simulink model "SF034A_AssiPahFwl"  (R2013b)
settings: Solver=FixedStepDiscrete  SolverMode=SingleTasking  StartTime=0.0  StopTime=1  FixedStep=0.002  RelTol=1e-3
values from neighbouring files (symbols this model uses):
  ARCHGLBPRM_2MILLISEC_SEC_F32 = DataDict.Constant    [SF034A_AssiPahFwl_DataDict.m]
  AssiPahFwlDiRcvr = DataDict.Calibration    [SF034A_AssiPahFwl_DataDict.m]
  AssiPahFwlHysCmpLim = DataDict.Calibration    [SF034A_AssiPahFwl_DataDict.m]
  AssiPahFwlRestoreThd = DataDict.Calibration    [SF034A_AssiPahFwl_DataDict.m]
  BasAssiPahFwlOverLimDiagcFailStep = DataDict.Calibration    [SF034A_AssiPahFwl_DataDict.m]
  BasAssiPahFwlOverLimDiagcPassStep = DataDict.Calibration    [SF034A_AssiPahFwl_DataDict.m]
  BASASSIREACHED_CNT_U08 = DataDict.Constant    [SF034A_AssiPahFwl_DataDict.m]
  HiFrqAssiPahFwlOverLimDiagcFailStep = DataDict.Calibration    [SF034A_AssiPahFwl_DataDict.m]
  HiFrqAssiPahFwlOverLimDiagcPassStep = DataDict.Calibration    [SF034A_AssiPahFwl_DataDict.m]
  HIFRQASSIREACHED_CNT_U08 = DataDict.Constant    [SF034A_AssiPahFwl_DataDict.m]
undefined symbols (not defined in the file or in its folder): MfgEnaSt1, NtcNr1, NtcSts1, sigbuilder_block, SigQlfr1
libraries: simulink x23, Fil x8, NxtrLim x5, FixdToFloat x5, BilnrIntrpnMplX x4, FloatToFixd x4, NxtrAbslt x2, LnrIntrpn x1, NxtrSign x1
(part 1 of 3)
settings Model: Creator=SNEHAP1  LastModifiedBy=PallavG
settings SolverCC: AutoInsertRateTranBlk=on  InsertRTBMode=Always
settings DataIOCC: LimitDataPoints=off  SaveFormat=Structure  ReturnWorkspaceOutputs=on
settings OptimizationCC: BlockReduction=off  InlineParams=on  ZeroExternalMemoryAtStartup=off  ZeroInternalMemoryAtStartup=off  OptimizeModelRefInitCode=on  LifeSpan=1
settings DebuggingCC: SignalInfNanChecking=error  SignalRangeChecking=warning  UnderspecifiedInitializationDetection=Simplified  SolverPrmCheckMsg=error  InheritedTsInSrcMsg=error  DiscreteInheritContinuousMsg=error  SingleTaskRateTransMsg=error  TasksWithSamePriorityMsg=error  SigSpecEnsureSampleTimeMsg=error  CheckMatrixSingularityMsg=error  ParameterUnderflowMsg=error  ParameterPrecisionLossMsg=error  ParameterTunabilityLossMsg=error  FixptConstUnderflowMsg=warning  FixptConstOverflowMsg=warning  VectorMatrixConversionMsg=error  SignalLabelMismatchMsg=error  UnconnectedInputMsg=error  UnconnectedOutputMsg=error  UnconnectedLineMsg=error  SFcnCompatibilityMsg=error  UniqueDataStoreMsg=warning  BusObjectLabelMismatch=error  RootOutportRequireBusObject=error  AssertControl=DisableAll  ModelReferenceIOMsg=error  ModelReferenceVersionMismatchMessage=warning  ModelReferenceIOMismatchMessage=error  ModelReferenceCSMismatchMessage=warning  ModelReferenceDataLoggingMessage=error  StateNameClashWarn=warning  StrictBusMsg=ErrorOnBusTreatedAsVector  NonBusSignalsTreatedAsBus=error  SFUnexpectedBacktrackingDiag=error  SFInvalidInputDataAccessInChartInitDiag=error  SFNoUnconditionalDefaultTransitionDiag=error  SFTransitionOutsideNaturalParentDiag=error  SFUnconditionalTransitionShadowingDiag=error  SFUndirectedBroadcastEventsDiag=error
settings ModelReferenceCC: ModelReferenceNumInstancesAllowed=Single
settings RTWCC: SystemTargetFile=autosar.tlc  GenCodeOnly=on  TemplateMakefile=ert_default_tmf  Description=AUTOSAR  GenerateReport=on  ProcessScript=autosar_make_rtw_hook  LaunchReport=on
settings CodeAppCC: GenerateComments=off  IgnoreCustomStorageClasses=off  CustomSymbolStrType=$N$R$M  CustomSymbolStrBlkIO=$N$M  SimulinkBlockComments=off
settings STFCustomTargetCC: ParMdlRefBuildCompliant=on  CompOptLevelCompliant=on  IncludeMdlTerminateFcn=off  CombineOutputUpdateFcns=on  SuppressErrorStatus=on  ERTFirstTimeCompliant=on  ERTCustomFileBanners=on  SupportNonFinite=off  SupportComplex=off  SupportContinuousTime=off  SupportNonInlinedSFcns=off  MATLABClassNameForMDSCustomization=Simulink.SoftwareTarget.ERTCustomization  AutosarCompliant=on  GRTInterface=off  SystemTargetFile=autosar.tlc
settings ERTTargetCC: CodeReplacementLibrary=ANSI_C  ConcurrentExecutionCompliant=off  IncludeMdlTerminateFcn=off  SuppressErrorStatus=on  SupportNonFinite=off  SupportComplex=off  ModelStepFunctionPrototypeControlCompliant=off  CPPClassGenCompliant=off  AutosarCompliant=on  InlinedParameterPlacement=NonHierarchical  ERTCustomFileTemplate=example_file_process.tlc  EnableUserReplacementTypes=on

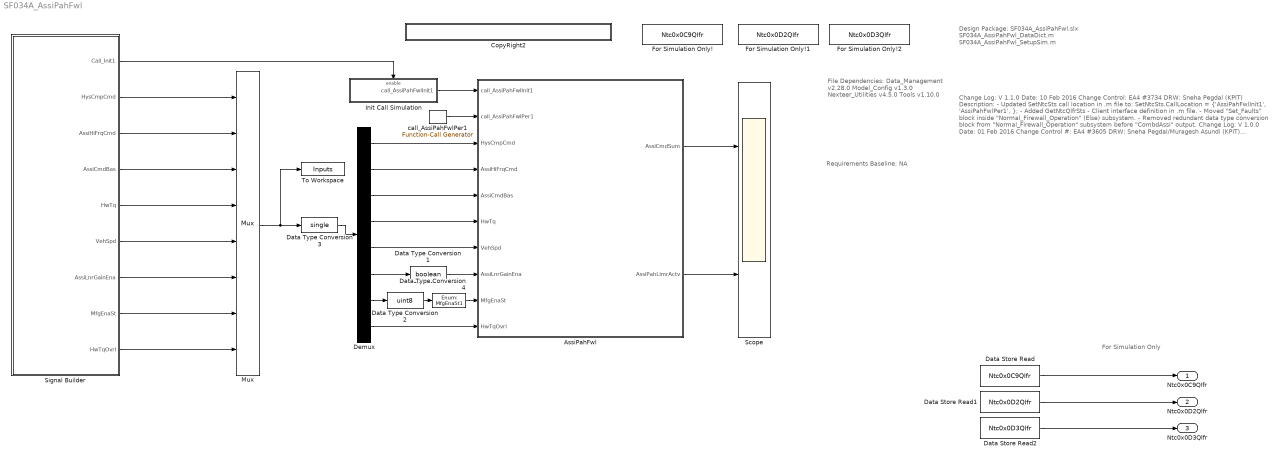
== system SF034A_AssiPahFwl ==
  note: Change Log:  V 1.1.0
      |  Date: 10 Feb 2016
      |  Change Control: EA4 #3734
      |  DRW: Sneha Pegdal (KPIT)
      |  Description:
      | - Updated SetNtcSts call location in .m file to:
      |   SetNtcSts.CallLocation = {'AssiPahFwlInit1', 'AssiPahFwlPer1', };
      | - Added GetNtcQlfrSts - Client interface definition in .m file.
      | - Moved "Set_Faults" block inside "Normal_Firewall_Operation" (Else) subsystem.
      | - Removed redundant data type conversion block from "Normal_Firewall_Operation" subsystem before
      |   "CombdAssi" output.
      |
      |
      |  Change Log:  V 1.0.0
      |  Date: 01 Feb 2016
      |  Change Control #: EA4 #3605
      |  DRW: Sneha Pegdal/Muragesh Asundi (KPIT)
      |  Description:
      |   -Initial Release of EA4 from EA3 V 10.0.0
  note: Requirements Baseline: NA
  note: For Simulation Only
  note: File Dependencies:
      |
      | Data_Management v2.28.0
      | Model_Config v1.3.0
      | Nexteer_Utilities v4.5.0
      | Tools v1.10.0
  note: Design Package:
      |
      | SF034A_AssiPahFwl.slx
      | SF034A_AssiPahFwl_DataDict.m
      | SF034A_AssiPahFwl_SetupSim.m
  AssiPahFwl : Subsystem
  CopyRight2 : Subsystem  Description=|  mask(Copyright Information){none=on}
      | Copyright info block.                                               
      |                                                                     
      | Place copyright information at the top of every subsystem in design.
      mask prompts: none "No parameters"
      mask help: Place copyright information at the top of every subsystem in design.
      mask Display:
      | NxtrConf = 'Nexteer Confidential';
      | 
      | sys = bdroot; %handle for the current model ("system")
      | first = get_param(sys,'Created');
      | first = first(end-3:end);  %year is last four digits
      | 
      | last = get_param(sys,'LastModifiedDate');
      | if isempty(last)
      |     last = datestr(now,'yyyy');
      | else
      |     last = last(end-3:end);
      | end
      | 
      | if strcmp(first,last)
      |     fprintf('%s -- Copyright %s Nexteer',NxtrConf,first)
      | else
      |     fprintf('%s -- %s%s- %s Nexteer',NxtrConf,char(169),first,last)
      | end
  Data Store Read : DataStoreRead  DataStoreName=Ntc0x0C9Qlfr  SampleTime=.002
  Data Store Read1 : DataStoreRead  DataStoreName=Ntc0x0D2Qlfr  SampleTime=.002
  Data Store Read2 : DataStoreRead  DataStoreName=Ntc0x0D3Qlfr  SampleTime=.002
  Data Type Conversion1 : DataTypeConversion  OutDataTypeStr=boolean
  Data Type Conversion2 : DataTypeConversion  OutDataTypeStr=uint8
  Data Type Conversion3 : DataTypeConversion  OutDataTypeStr=single
  Data Type Conversion4 : DataTypeConversion  OutDataTypeStr=Enum: MfgEnaSt1
  Demux : Demux  Outputs=8
  For Simulation Only! : DataStoreMemory  DataStoreName=Ntc0x0C9Qlfr  InitialValue=SigQlfr1.SIGQLFR_NORES  OutDataTypeStr=Enum: SigQlfr1
  For Simulation Only!1 : DataStoreMemory  DataStoreName=Ntc0x0D2Qlfr  InitialValue=SigQlfr1.SIGQLFR_NORES  OutDataTypeStr=Enum: SigQlfr1
  For Simulation Only!2 : DataStoreMemory  DataStoreName=Ntc0x0D3Qlfr  InitialValue=SigQlfr1.SIGQLFR_NORES  OutDataTypeStr=Enum: SigQlfr1
  Init Call Simulation : Subsystem  TreatAsAtomicUnit=on
  Mux : Mux  Inputs=8
  Scope : Scope  NumInputPorts=2
      settings: YMin=-5~-5  YMax=5~5
  Signal Builder : Subsystem  Tag=STV Subsys  LoadFcn=sigbuilder_block('load');  StartFcn=sigbuilder_block('start');  StopFcn=sigbuilder_block('stop');  ClipboardFcn=sigbuilder_block('clipboard');  mask(Sigbuilder block){}
      mask help: Simulink:masks:SigbuilderBlock_MD
      mask init:
      | if ~strcmp(get_param(bdroot(gcbh),'SimulationStatus'),'stopped') tuvar = sigbuilder_block('maskInit'); end
      settings: CopyFcn=sigbuilder_block('copy');  DeleteFcn=sigbuilder_block('delete');  ModelCloseFcn=sigbuilder_block('modelClose');  PreSaveFcn=sigbuilder_block('preSave');  PauseFcn=sigbuilder_block('pause');  ContinueFcn=sigbuilder_block('continue');  NameChangeFcn=sigbuilder_block('namechange');  OpenFcn=sigbuilder_block('open',[6 28.5 756 480 ]);  CloseFcn=sigbuilder_block('close');
      mask Display: plot(0, 0, 100, 100,[2, 2, 32, 32, 2], [68, 8, 8, 68, 68],[32, 2], [38, 38], [32, 19, 2],[53, 60, 44], [32, 17, 17, 2],[16, 16, 31, 31]);txt = getActiveGroup(gcbh);text(2, 100, txt,'verticalAlignment', 'top');
  To Workspace : ToWorkspace  VariableName=Inputs  SampleTime=-1
  call_AssiPahFwlPer1 : simulink/Ports & Subsystems/Function-Call Generator  RequirementInfo={} %GIDa_9fbb524b_78b2_48c0_ad45_2c0b0cc0a9b8  sample_time=0.002  numberOfIterations=1
  Ntc0x0C9Qlfr : Outport
  Ntc0x0D2Qlfr : Outport  Port=2
  Ntc0x0D3Qlfr : Outport  Port=3
  wires:
  call_AssiPahFwlPer1/1 -> AssiPahFwl/2(call_AssiPahFwlPer1)
  Data Store Read/1 -> Ntc0x0C9Qlfr/1
  Data Store Read1/1 -> Ntc0x0D2Qlfr/1
  Data Store Read2/1 -> Ntc0x0D3Qlfr/1
  Mux/1 -> Data Type Conversion3/1, To Workspace/1
  Init Call Simulation/1(call_AssiPahFwlInit1) -> AssiPahFwl/1(call_AssiPahFwlInit1)
  Demux/3 -> AssiPahFwl/5(AssiCmdBas)
  Demux/4 -> AssiPahFwl/6(HwTq)
  Demux/2 -> AssiPahFwl/4(AssiHiFrqCmd)
  Demux/5 -> AssiPahFwl/7(VehSpd)
  Demux/1 -> AssiPahFwl/3(HysCmpCmd)
  Demux/7 -> Data Type Conversion2/1
  Demux/8 -> AssiPahFwl/10(HwTqOvrl)
  AssiPahFwl/1(AssiCmdSum) -> Scope/1
  AssiPahFwl/2(AssiPahLimrActv) -> Scope/2
  Signal Builder/1(Call_Init1) -> Init Call Simulation/Enable
  Signal Builder/2(HysCmpCmd) -> Mux/1
  Signal Builder/3(AssiHiFrqCmd) -> Mux/2
  Signal Builder/4(AssiCmdBas) -> Mux/3
  Signal Builder/5(HwTq) -> Mux/4
  Signal Builder/6(VehSpd) -> Mux/5
  Signal Builder/7(AssiLnrGainEna) -> Mux/6
  Signal Builder/8(MfgEnaSt) -> Mux/7
  Signal Builder/9(HwTqOvrl) -> Mux/8
  Data Type Conversion3/1 -> Demux/1
  Demux/6 -> Data Type Conversion1/1
  Data Type Conversion1/1 -> AssiPahFwl/8(AssiLnrGainEna)
  Data Type Conversion2/1 -> Data Type Conversion4/1
  Data Type Conversion4/1 -> AssiPahFwl/9(MfgEnaSt)

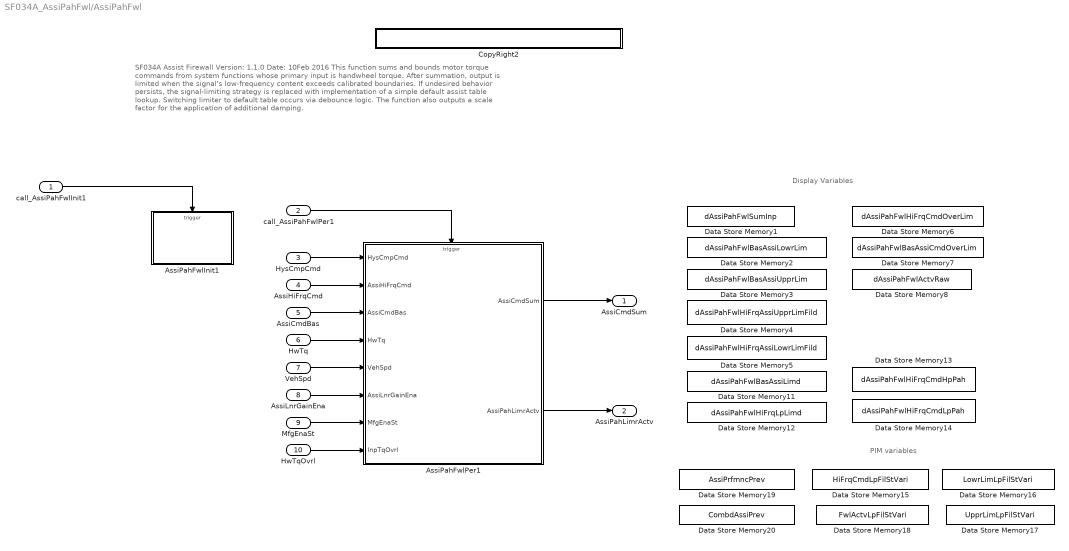
== system SF034A_AssiPahFwl/AssiPahFwl ==
  note: Display Variables
  note: SF034A Assist Firewall
      | Version: 1.1.0                                                                                                                                                                                           Date: 10Feb 2016
      |
      | This function sums and bounds motor torque commands from system functions whose primary input is handwheel torque.
      | After summation, output is limited when the signal's low-frequency content
      | exceeds calibrated boundaries.  If undesired behavior persists,  the signal-limiting strategy is replaced with implementation of a simple default assist table lookup.
      | Switching limiter to default table occurs via debounce logic.  The function also outputs a scale factor for the application of additional damping.
  note: PIM variables
  call_AssiPahFwlInit1 : Inport
  call_AssiPahFwlPer1 : Inport  Port=2
  HysCmpCmd : Inport  Port=3
  AssiHiFrqCmd : Inport  Port=4
  AssiCmdBas : Inport  Port=5
  HwTq : Inport  Port=6
  VehSpd : Inport  Port=7
  AssiLnrGainEna : Inport  Port=8
  MfgEnaSt : Inport  Port=9
  HwTqOvrl : Inport  Port=10
  AssiPahFwlInit1 : Subsystem  TreatAsAtomicUnit=on
  AssiPahFwlPer1 : Subsystem
  CopyRight2 : Subsystem  Description=|  mask(Copyright Information){none=on}
      | Copyright info block.                                               
      |                                                                     
      | Place copyright information at the top of every subsystem in design.
      mask prompts: none "No parameters"
      mask help: Place copyright information at the top of every subsystem in design.
      mask Display:
      | NxtrConf = 'Nexteer Confidential';
      | 
      | sys = bdroot; %handle for the current model ("system")
      | first = get_param(sys,'Created');
      | first = first(end-3:end);  %year is last four digits
      | 
      | last = get_param(sys,'LastModifiedDate');
      | if isempty(last)
      |     last = datestr(now,'yyyy');
      | else
      |     last = last(end-3:end);
      | end
      | 
      | if strcmp(first,last)
      |     fprintf('%s -- Copyright %s Nexteer',NxtrConf,first)
      | else
      |     fprintf('%s -- %s%s- %s Nexteer',NxtrConf,char(169),first,last)
      | end
  Data Store Memory1 : DataStoreMemory  DataStoreName=dAssiPahFwlSumInp  StateMustResolveToSignalObject=on
  Data Store Memory11 : DataStoreMemory  DataStoreName=dAssiPahFwlBasAssiLimd  OutDataTypeStr=single  StateMustResolveToSignalObject=on
  Data Store Memory12 : DataStoreMemory  DataStoreName=dAssiPahFwlHiFrqLpLimd  OutDataTypeStr=single  StateMustResolveToSignalObject=on
  Data Store Memory13 : DataStoreMemory  DataStoreName=dAssiPahFwlHiFrqCmdHpPah  OutDataTypeStr=single  StateMustResolveToSignalObject=on
  Data Store Memory14 : DataStoreMemory  DataStoreName=dAssiPahFwlHiFrqCmdLpPah  OutDataTypeStr=single  StateMustResolveToSignalObject=on
  Data Store Memory15 : DataStoreMemory  DataStoreName=HiFrqCmdLpFilStVari  InitialValue=[]  OutDataTypeStr=Bus: FilLpRec1  StateMustResolveToSignalObject=on
  Data Store Memory16 : DataStoreMemory  DataStoreName=LowrLimLpFilStVari  InitialValue=[]  OutDataTypeStr=Bus: FilLpRec1  StateMustResolveToSignalObject=on
  Data Store Memory17 : DataStoreMemory  DataStoreName=UpprLimLpFilStVari  InitialValue=[]  OutDataTypeStr=Bus: FilLpRec1  StateMustResolveToSignalObject=on
  Data Store Memory18 : DataStoreMemory  DataStoreName=FwlActvLpFilStVari  InitialValue=[]  OutDataTypeStr=Bus: FilLpRec1  StateMustResolveToSignalObject=on
  Data Store Memory19 : DataStoreMemory  DataStoreName=AssiPrfmncPrev  StateMustResolveToSignalObject=on
  Data Store Memory2 : DataStoreMemory  DataStoreName=dAssiPahFwlBasAssiLowrLim  OutDataTypeStr=single  StateMustResolveToSignalObject=on
  Data Store Memory20 : DataStoreMemory  DataStoreName=CombdAssiPrev  StateMustResolveToSignalObject=on
  Data Store Memory3 : DataStoreMemory  DataStoreName=dAssiPahFwlBasAssiUpprLim  OutDataTypeStr=single  StateMustResolveToSignalObject=on
  Data Store Memory4 : DataStoreMemory  DataStoreName=dAssiPahFwlHiFrqAssiUpprLimFild  OutDataTypeStr=single  StateMustResolveToSignalObject=on
  Data Store Memory5 : DataStoreMemory  DataStoreName=dAssiPahFwlHiFrqAssiLowrLimFild  OutDataTypeStr=single  StateMustResolveToSignalObject=on
  Data Store Memory6 : DataStoreMemory  DataStoreName=dAssiPahFwlHiFrqCmdOverLim  OutDataTypeStr=boolean  StateMustResolveToSignalObject=on
  Data Store Memory7 : DataStoreMemory  DataStoreName=dAssiPahFwlBasAssiCmdOverLim  OutDataTypeStr=boolean  StateMustResolveToSignalObject=on
  Data Store Memory8 : DataStoreMemory  DataStoreName=dAssiPahFwlActvRaw  OutDataTypeStr=single  StateMustResolveToSignalObject=on
  AssiCmdSum : Outport
  AssiPahLimrActv : Outport  Port=2
  wires:
  AssiPahFwlPer1/1(AssiCmdSum) -> AssiCmdSum/1
  AssiPahFwlPer1/2(AssiPahLimrActv) -> AssiPahLimrActv/1
  call_AssiPahFwlPer1/1 -> AssiPahFwlPer1/Trigger
  HysCmpCmd/1 -> AssiPahFwlPer1/1(HysCmpCmd)
  AssiHiFrqCmd/1 -> AssiPahFwlPer1/2(AssiHiFrqCmd)
  AssiCmdBas/1 -> AssiPahFwlPer1/3(AssiCmdBas)
  VehSpd/1 -> AssiPahFwlPer1/5(VehSpd)
  HwTq/1 -> AssiPahFwlPer1/4(HwTq)
  AssiLnrGainEna/1 -> AssiPahFwlPer1/6(AssiLnrGainEna)
  MfgEnaSt/1 -> AssiPahFwlPer1/7(MfgEnaSt)
  HwTqOvrl/1 -> AssiPahFwlPer1/8(InpTqOvrl)
  call_AssiPahFwlInit1/1 -> AssiPahFwlInit1/Trigger

== system SF034A_AssiPahFwl/CopyRight2 ==

== system SF034A_AssiPahFwl/Init Call Simulation ==
  Enable : EnablePort
  CopyRight2 : Subsystem  Description=|  mask(Copyright Information){none=on}
      | Copyright info block.                                               
      |                                                                     
      | Place copyright information at the top of every subsystem in design.
      mask prompts: none "No parameters"
      mask help: Place copyright information at the top of every subsystem in design.
      mask Display:
      | NxtrConf = 'Nexteer Confidential';
      | 
      | sys = bdroot; %handle for the current model ("system")
      | first = get_param(sys,'Created');
      | first = first(end-3:end);  %year is last four digits
      | 
      | last = get_param(sys,'LastModifiedDate');
      | if isempty(last)
      |     last = datestr(now,'yyyy');
      | else
      |     last = last(end-3:end);
      | end
      | 
      | if strcmp(first,last)
      |     fprintf('%s -- Copyright %s Nexteer',NxtrConf,first)
      | else
      |     fprintf('%s -- %s%s- %s Nexteer',NxtrConf,char(169),first,last)
      | end
  call_AssiPahFwlInit : simulink/Ports & Subsystems/Function-Call Generator  RequirementInfo={} %GIDa_1b7e385f_3d84_4186_97bf_20680bb5493f  sample_time=0  numberOfIterations=1
  call_AssiPahFwlInit1 : Outport
  wires:
  call_AssiPahFwlInit/1 -> call_AssiPahFwlInit1/1

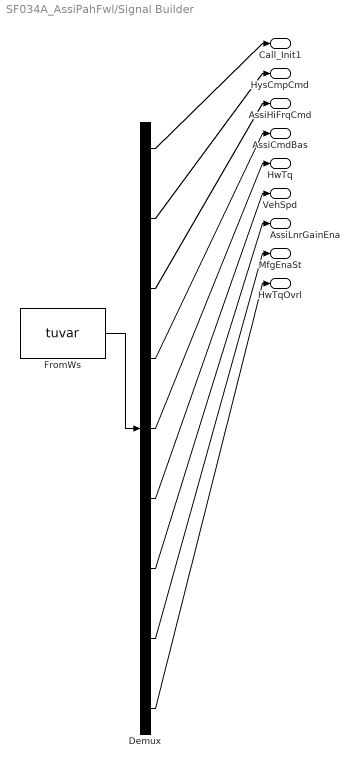
== system SF034A_AssiPahFwl/Signal Builder ==
  Demux : Demux  Tag=STV Demux  Outputs=9
  FromWs : FromWorkspace  Tag=STV FromWs  VariableName=tuvar  SampleTime=0
      SigBuilderData=|
      | common.afterFinalStr = 'Extrapolate'
      | common.sampleTime = 0
      | dataSet.timeRange = [0 0.31]
      | dataSet.name = 'TestCase_1'
      | sbobj.Name = 'Signal Builder'
      | sbobj.Groups.Name = 'TestCase_1'
      | sbobj.Groups.Signals(1).Name = 'Call_Init1'
      | sbobj.Groups.Signals(1).XData = [0 0.002 0.004 0.006 0.008 0.01 0.012 0.014 0.016 0.018 0.02 0.022 0.024 0.026 0.028 0.03 0.032 0.034 0.036 0.038 0.04 0.042 0.044 0.046 0.048 0.05 0.052 0.054 0.056 0.058 0.06 0.062 0.064 0.066 0.068 0.07 0.072 0.074 0.076 0.078 0.08 0.082 0.084 0.086 0.088 0.09 0.092 0.094 0.096 0.098 0.1 0.102 0.104 0.106 0.108 0.11 0.112 0.114 0.116 0.118 0.12 0.122 0.124 0.126 0.128 0.13 0.132 0.134 0.136 0.138 0.14 0.142 0.144 0.146 0.148 0.15 0.152 0.154 0.156 0.158 0.16 0.162 0.164 0.166 0.168 0.17 0.172 0.174 0.176 0.178 0.18 0.182 0.184 0.186 0.188 0.19 0.192 0.194 0.196 0.198 0.2 0.202 0.204 0.206 0.208 0.21 0.212 0.214 0.216 0.218 0.22 0.222 0.224 0.226 0.228 0.23 0.232 0.234 0.236 0.238 0.24 0.242 0.244 0.246 0.248 0.25 0.252 0.254 0.256 0.258 0.26 0.262 0.264 0.266 0.268 0.27 0.272 0.274 0.276 0.278 0.28 0.282 0.284 0.286 0.288 0.29 0.292 0.294 0.296 0.298 0.3 0.302 0.304 0.306 0.308 0.31]
      | sbobj.Groups.Signals(1).YData = [1 0 0 0 0 0 0 0 0 0 0 0 0 0 0 0 0 0 0 0 0 0 0 0 0 0 0 0 0 0 0 0 0 0 0 0 0 0 0 0 0 0 0 0 0 0 0 0 0 0 0 0 0 0 0 0 0 0 0 0 0 0 0 0 0 0 0 0 0 0 0 0 0 0 0 0 0 0 0 0 0 0 0 0 0 0 0 0 0 0 0 0 0 0 0 0 0 0 0 0 0 0 0 0 0 0 0 0 0 0 0 0 0 0 0 0 0 0 0 0 0 0 0 0 0 0 0 0 0 0 0 0 0 0 0 0 0 0 0 0 0 0 0 0 0 0 0 0 0 0 0 0 0 0 0 0]
      | sbobj.Groups.Signals(2).Name = 'HysCmpCmd'
      | sbobj.Groups.Signals(2).XData = [0 0.002 0.004 0.006 0.008 0.01 0.012 0.014 0.016 0.018 0.02 0.022 0.024 0.026 0.028 0.03 0.032 0.034 0.036 0.038 0.04 0.042 0.044 0.046 0.048 0.05 0.052 0.054 0.056 0.058 0.06 0.062 0.064 0.066 0.068 0.07 0.072 0.074 0.076 0.078 0.08 0.082 0.084 0.086 0.088 0.09 0.092 0.094 0.096 0.098 0.1 0.102 0.104 0.106 0.108 0.11 0.112 0.114 0.116 0.118 0.12 0.122 0.124 0.126 0.128 0.13 0.132 0.134 0.136 0.138 0.14 0.142 0.144 0.146 0.148 0.15 0.152 0.154 0.156 0.158 0.16 0.162 0.164 0.166 0.168 0.17 0.172 0.174 0.176 0.178 0.18 0.182 0.184 0.186 0.188 0.19 0.192 0.194 0.196 0.198 0.2 0.202 0.204 0.206 0.208 0.21 0.212 0.214 0.216 0.218 0.22 0.222 0.224 0.226 0.228 0.23 0.232 0.234 0.236 0.238 0.24 0.242 0.244 0.246 0.248 0.25 0.252 0.254 0.256 0.258 0.26 0.262 0.264 0.266 0.268 0.27 0.272 0.274 0.276 0.278 0.28 0.282 0.284 0.286 0.288 0.29 0.292 0.294 0.296 0.298 0.3 0.302 0.304 0.306 0.308 0.31]
      | sbobj.Groups.Signals(2).YData = [0 0.736365021324 1.4675649711 2.18847100705 2.8940264913 3.57928245907 4.2394323321 4.86984563334 5.46610046645 6.02401453217 6.5396744642 7.00946327861 ... (156 elements, 1x156)]
      | sbobj.Groups.Signals(3).Name = 'AssiHiFrqCmd'
      | sbobj.Groups.Signals(3).XData = [0 0.002 0.004 0.006 0.008 0.01 0.012 0.014 0.016 0.018 0.02 0.022 0.024 0.026 0.028 0.03 0.032 0.034 0.036 0.038 0.04 0.042 0.044 0.046 0.048 0.05 0.052 0.054 0.056 0.058 0.06 0.062 0.064 0.066 0.068 0.07 0.072 0.074 0.076 0.078 0.08 0.082 0.084 0.086 0.088 0.09 0.092 0.094 0.096 0.098 0.1 0.102 0.104 0.106 0.108 0.11 0.112 0.114 0.116 0.118 0.12 0.122 0.124 0.126 0.128 0.13 0.132 0.134 0.136 0.138 0.14 0.142 0.144 0.146 0.148 0.15 0.152 0.154 0.156 0.158 0.16 0.162 0.164 0.166 0.168 0.17 0.172 0.174 0.176 0.178 0.18 0.182 0.184 0.186 0.188 0.19 0.192 0.194 0.196 0.198 0.2 0.202 0.204 0.206 0.208 0.21 0.212 0.214 0.216 0.218 0.22 0.222 0.224 0.226 0.228 0.23 0.232 0.234 0.236 0.238 0.24 0.242 0.244 0.246 0.248 0.25 0.252 0.254 0.256 0.258 0.26 0.262 0.264 0.266 0.268 0.27 0.272 0.274 0.276 0.278 0.28 0.282 0.284 0.286 0.288 0.29 0.292 0.294 0.296 0.298 0.3 0.302 0.304 0.306 0.308 0.31]
      | sbobj.Groups.Signals(3).YData = [8.8 8.75179267924 8.64412780641 8.47583058782 8.24808150753 7.9624780617 7.6210235533 7.22611304038 6.78051653643 6.28735958077 5.75010131511 5.17251022017 ... (156 elements, 1x156)]
      | sbobj.Groups.Signals(4).Name = 'AssiCmdBas'
      | sbobj.Groups.Signals(4).XData = [0 0.002 0.004 0.006 0.008 0.01 0.012 0.014 0.016 0.018 0.02 0.022 0.024 0.026 0.028 0.03 0.032 0.034 0.036 0.038 0.04 0.042 0.044 0.046 0.048 0.05 0.052 0.054 0.056 0.058 0.06 0.062 0.064 0.066 0.068 0.07 0.072 0.074 0.076 0.078 0.08 0.082 0.084 0.086 0.088 0.09 0.092 0.094 0.096 0.098 0.1 0.102 0.104 0.106 0.108 0.11 0.112 0.114 0.116 0.118 0.12 0.122 0.124 0.126 0.128 0.13 0.132 0.134 0.136 0.138 0.14 0.142 0.144 0.146 0.148 0.15 0.152 0.154 0.156 0.158 0.16 0.162 0.164 0.166 0.168 0.17 0.172 0.174 0.176 0.178 0.18 0.182 0.184 0.186 0.188 0.19 0.192 0.194 0.196 0.198 0.2 0.202 0.204 0.206 0.208 0.21 0.212 0.214 0.216 0.218 0.22 0.222 0.224 0.226 0.228 0.23 0.232 0.234 0.236 0.238 0.24 0.242 0.244 0.246 0.248 0.25 0.252 0.254 0.256 0.258 0.26 0.262 0.264 0.266 0.268 0.27 0.272 0.274 0.276 0.278 0.28 0.282 0.284 0.286 0.288 0.29 0.292 0.294 0.296 0.298 0.3 0.302 0.304 0.306 0.308 0.31]
      | sbobj.Groups.Signals(4).YData = [-8.8 -8.78263521017 -8.70559653007 -8.56749434528 -8.3692973434 -8.11239573398 -7.79859149723 -7.43008574442 -7.00946327861 -6.5396744642 -6.02401453217 -5.46610046645 ... (156 elements, 1x156)]
      | sbobj.Groups.Signals(5).Name = 'HwTq'
      | sbobj.Groups.Signals(5).XData = [0 0.002 0.004 0.006 0.008 0.01 0.012 0.014 0.016 0.018 0.02 0.022 0.024 0.026 0.028 0.03 0.032 0.034 0.036 0.038 0.04 0.042 0.044 0.046 0.048 0.05 0.052 0.054 0.056 0.058 0.06 0.062 0.064 0.066 0.068 0.07 0.072 0.074 0.076 0.078 0.08 0.082 0.084 0.086 0.088 0.09 0.092 0.094 0.096 0.098 0.1 0.102 0.104 0.106 0.108 0.11 0.112 0.114 0.116 0.118 0.12 0.122 0.124 0.126 0.128 0.13 0.132 0.134 0.136 0.138 0.14 0.142 0.144 0.146 0.148 0.15 0.152 0.154 0.156 0.158 0.16 0.162 0.164 0.166 0.168 0.17 0.172 0.174 0.176 0.178 0.18 0.182 0.184 0.186 0.188 0.19 0.192 0.194 0.196 0.198 0.2 0.202 0.204 0.206 0.208 0.21 0.212 0.214 0.216 0.218 0.22 0.222 0.224 0.226 0.228 0.23 0.232 0.234 0.236 0.238 0.24 0.242 0.244 0.246 0.248 0.25 0.252 0.254 0.256 0.258 0.26 0.262 0.264 0.266 0.268 0.27 0.272 0.274 0.276 0.278 0.28 0.282 0.284 0.286 0.288 0.29 0.292 0.294 0.296 0.298 0.3 0.302 0.304 0.306 0.308 0.31]
      | sbobj.Groups.Signals(5).YData = [0 0.418756537292 0.836778433323 1.25333233564 1.66768746716 2.07911690818 2.48689887165 2.89031796944 3.28866646739 3.68124552685 4.06736643076 4.44635179185 ... (156 elements, 1x156)]
      | sbobj.Groups.Signals(6).Name = 'VehSpd'
      | sbobj.Groups.Signals(6).XData = [0 0.002 0.004 0.006 0.008 0.01 0.012 0.014 0.016 0.018 0.02 0.022 0.024 0.026 0.028 0.03 0.032 0.034 0.036 0.038 0.04 0.042 0.044 0.046 0.048 0.05 0.052 0.054 0.056 0.058 0.06 0.062 0.064 0.066 0.068 0.07 0.072 0.074 0.076 0.078 0.08 0.082 0.084 0.086 0.088 0.09 0.092 0.094 0.096 0.098 0.1 0.102 0.104 0.106 0.108 0.11 0.112 0.114 0.116 0.118 0.12 0.122 0.124 0.126 0.128 0.13 0.132 0.134 0.136 0.138 0.14 0.142 0.144 0.146 0.148 0.15 0.152 0.154 0.156 0.158 0.16 0.162 0.164 0.166 0.168 0.17 0.172 0.174 0.176 0.178 0.18 0.182 0.184 0.186 0.188 0.19 0.192 0.194 0.196 0.198 0.2 0.202 0.204 0.206 0.208 0.21 0.212 0.214 0.216 0.218 0.22 0.222 0.224 0.226 0.228 0.23 0.232 0.234 0.236 0.238 0.24 0.242 0.244 0.246 0.248 0.25 0.252 0.254 0.256 0.258 0.26 0.262 0.264 0.266 0.268 0.27 0.272 0.274 0.276 0.278 0.28 0.282 0.284 0.286 0.288 0.29 0.292 0.294 0.296 0.298 0.3 0.302 0.304 0.306 0.308 0.31]
      | sbobj.Groups.Signals(6).YData = [0 21.3984590556 42.7593779428 64.0452823514 85.2188295719 106.242874008 127.080532341 147.695248239 168.050856483 188.111646422 207.842424612 227.208576563 ... (156 elements, 1x156)]
      | sbobj.Groups.Signals(7).Name = 'AssiLnrGainEna'
      | sbobj.Groups.Signals(7).XData = [0 0.002 0.004 0.006 0.008 0.01 0.012 0.014 0.016 0.018 0.02 0.022 0.024 0.026 0.028 0.03 0.032 0.034 0.036 0.038 0.04 0.042 0.044 0.046 0.048 0.05 0.052 0.054 0.056 0.058 0.06 0.062 0.064 0.066 0.068 0.07 0.072 0.074 0.076 0.078 0.08 0.082 0.084 0.086 0.088 0.09 0.092 0.094 0.096 0.098 0.1 0.102 0.104 0.106 0.108 0.11 0.112 0.114 0.116 0.118 0.12 0.122 0.124 0.126 0.128 0.13 0.132 0.134 0.136 0.138 0.14 0.142 0.144 0.146 0.148 0.15 0.152 0.154 0.156 0.158 0.16 0.162 0.164 0.166 0.168 0.17 0.172 0.174 0.176 0.178 0.18 0.182 0.184 0.186 0.188 0.19 0.192 0.194 0.196 0.198 0.2 0.202 0.204 0.206 0.208 0.21 0.212 0.214 0.216 0.218 0.22 0.222 0.224 0.226 0.228 0.23 0.232 0.234 0.236 0.238 0.24 0.242 0.244 0.246 0.248 0.25 0.252 0.254 0.256 0.258 0.26 0.262 0.264 0.266 0.268 0.27 0.272 0.274 0.276 0.278 0.28 0.282 0.284 0.286 0.288 0.29 0.292 0.294 0.296 0.298 0.3 0.302 0.304 0.306 0.308 0.31]
      | sbobj.Groups.Signals(7).YData = [0 0 0 0 0 0 0 0 0 0 0 0 0 0 0 0 0 0 0 0 0 0 0 0 0 0 0 0 0 0 0 0 0 0 0 0 0 0 0 0 0 0 0 0 0 0 0 0 0 0 0 0 0 0 0 0 0 0 0 0 0 0 0 0 0 0 0 0 0 0 0 0 0 0 0 0 1 1 1 1 1 1 1 1 1 1 1 1 1 1 1 1 1 1 1 1 1 1 1 1 1 1 1 1 1 1 1 1 1 1 1 1 1 1 1 1 1 1 1 1 1 1 1 1 1 1 1 1 1 1 1 1 1 1 1 1 1 1 1 1 1 1 1 1 1 1 1 1 1 1 1 1 1 1 1 1]
      | sbobj.Groups.Signals(8).Name = 'MfgEnaSt'
      | sbobj.Groups.Signals(8).XData = [0 0.002 0.004 0.006 0.008 0.01 0.012 0.014 0.016 0.018 0.02 0.022 0.024 0.026 0.028 0.03 0.032 0.034 0.036 0.038 0.04 0.042 0.044 0.046 0.048 0.05 0.052 0.054 0.056 0.058 0.06 0.062 0.064 0.066 0.068 0.07 0.072 0.074 0.076 0.078 0.08 0.082 0.084 0.086 0.088 0.09 0.092 0.094 0.096 0.098 0.1 0.102 0.104 0.106 0.108 0.11 0.112 0.114 0.116 0.118 0.12 0.122 0.124 0.126 0.128 0.13 0.132 0.134 0.136 0.138 0.14 0.142 0.144 0.146 0.148 0.15 0.152 0.154 0.156 0.158 0.16 0.162 0.164 0.166 0.168 0.17 0.172 0.174 0.176 0.178 0.18 0.182 0.184 0.186 0.188 0.19 0.192 0.194 0.196 0.198 0.2 0.202 0.204 0.206 0.208 0.21 0.212 0.214 0.216 0.218 0.22 0.222 0.224 0.226 0.228 0.23 0.232 0.234 0.236 0.238 0.24 0.242 0.244 0.246 0.248 0.25 0.252 0.254 0.256 0.258 0.26 0.262 0.264 0.266 0.268 0.27 0.272 0.274 0.276 0.278 0.28 0.282 0.284 0.286 0.288 0.29 0.292 0.294 0.296 0.298 0.3 0.302 0.304 0.306 0.308 0.31]
      | sbobj.Groups.Signals(8).YData = [0 0 0 2 2 2 2 2 2 2 2 2 2 2 2 2 2 2 2 2 2 2 2 2 2 2 2 2 2 2 2 2 2 2 2 2 2 2 2 2 2 2 2 2 2 2 2 2 2 2 2 2 2 2 2 2 2 2 2 2 2 2 2 2 2 2 2 2 2 2 2 2 2 2 2 3.12284933783e-14 0 2 2 2 2 2 2 2 2 2 2 2 2 2 2 2 2 2 2 2 2 2 2 2 2 2 2 2 2 2 2 2 2 2 2 2 2 2 2 2 2 2 2 2 2 2 2 2 2 2 2 2 2 2 2 2 2 2 2 2 2 2 2 2 2 2 2 2 2 2 2 2 2 2 2 3.12284933783e-14 0 2 2 2]
      | sbobj.Groups.Signals(9).Name = 'HwTqOvrl'
      | sbobj.Groups.Signals(9).XData = [0 0.002 0.004 0.006 0.008 0.01 0.012 0.014 0.016 0.018 0.02 0.022 0.024 0.026 0.028 0.03 0.032 0.034 0.036 0.038 0.04 0.042 0.044 0.046 0.048 0.05 0.052 0.054 0.056 0.058 0.06 0.062 0.064 0.066 0.068 0.07 0.072 0.074 0.076 0.078 0.08 0.082 0.084 0.086 0.088 0.09 0.092 0.094 0.096 0.098 0.1 0.102 0.104 0.106 0.108 0.11 0.112 0.114 0.116 0.118 0.12 0.122 0.124 0.126 0.128 0.13 0.132 0.134 0.136 0.138 0.14 0.142 0.144 0.146 0.148 0.15 0.152 0.154 0.156 0.158 0.16 0.162 0.164 0.166 0.168 0.17 0.172 0.174 0.176 0.178 0.18 0.182 0.184 0.186 0.188 0.19 0.192 0.194 0.196 0.198 0.2 0.202 0.204 0.206 0.208 0.21 0.212 0.214 0.216 0.218 0.22 0.222 0.224 0.226 0.228 0.23 0.232 0.234 0.236 0.238 0.24 0.242 0.244 0.246 0.248 0.25 0.252 0.254 0.256 0.258 0.26 0.262 0.264 0.266 0.268 0.27 0.272 0.274 0.276 0.278 0.28 0.282 0.284 0.286 0.288 0.29 0.292 0.294 0.296 0.298 0.3 0.302 0.304 0.306 0.308 0.31]
      | sbobj.Groups.Signals(9).YData = [0 0.314107590781 0.627905195293 0.941083133185 1.25333233564 1.5643446504 1.87381314586 2.18143241397 2.48689887165 2.78991106039 3.09016994375 3.38737920245 ... (156 elements, 1x156)]
      | sbobj.Groups.TimeRange = [0 0.31]
  Call_Init1 : Outport
  HysCmpCmd : Outport  Tag=STV Outport  Port=2
  AssiHiFrqCmd : Outport  Tag=STV Outport  Port=3
  AssiCmdBas : Outport  Tag=STV Outport  Port=4
  HwTq : Outport  Tag=STV Outport  Port=5
  VehSpd : Outport  Tag=STV Outport  Port=6
  AssiLnrGainEna : Outport  Tag=STV Outport  Port=7
  MfgEnaSt : Outport  Tag=STV Outport  Port=8
  HwTqOvrl : Outport  Tag=STV Outport  Port=9
  wires:
  FromWs/1 -> Demux/1
  Demux/1 -> Call_Init1/1
  Demux/2 -> HysCmpCmd/1
  Demux/3 -> AssiHiFrqCmd/1
  Demux/4 -> AssiCmdBas/1
  Demux/5 -> HwTq/1
  Demux/6 -> VehSpd/1
  Demux/7 -> AssiLnrGainEna/1
  Demux/8 -> MfgEnaSt/1
  Demux/9 -> HwTqOvrl/1

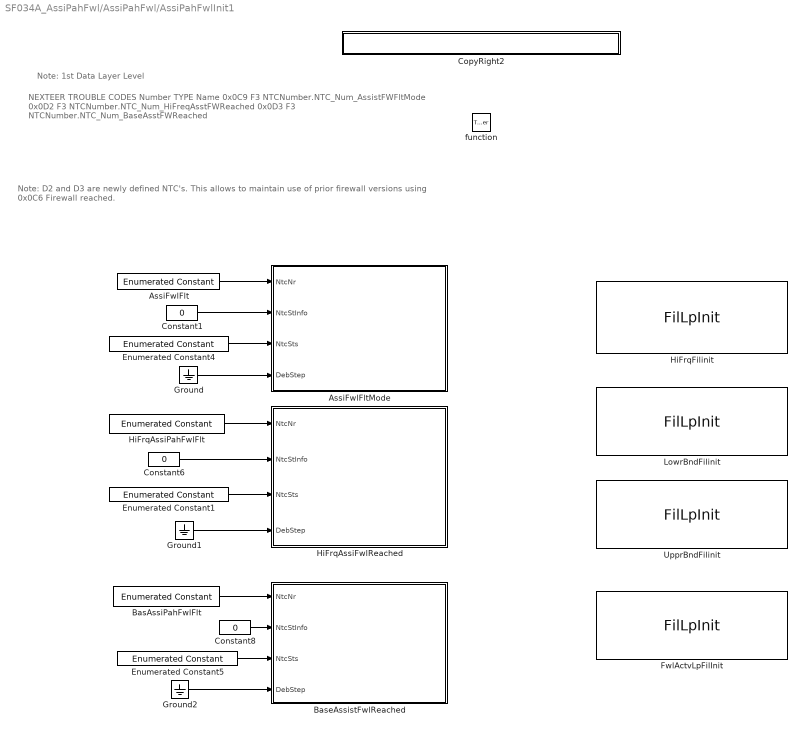
== system SF034A_AssiPahFwl/AssiPahFwl/AssiPahFwlInit1 ==
  note: Note: 1st Data Layer Level
  note: Note: D2 and D3 are newly defined NTC's.  This allows to maintain use of prior firewall versions using
      |  0x0C6 Firewall reached.
  note: NEXTEER TROUBLE CODES
      | Number  TYPE   Name
      |  0x0C9      F3      NTCNumber.NTC_Num_AssistFWFltMode
      |  0x0D2      F3      NTCNumber.NTC_Num_HiFreqAsstFWReached
      |  0x0D3      F3      NTCNumber.NTC_Num_BaseAsstFWReached
  function : TriggerPort  TriggerType=function-call
  AssiFwlFlt : simulink/Sources/Enumerated Constant  RequirementInfo={} %GIDa_c8c75cce_4fec_4ec0_9a78_eab890d1076a  OutDataTypeStr=Enum: NtcNr1  Value=NtcNr1.NTCNR_0X0C9  SampleTime=inf
  AssiFwlFltMode : Subsystem  RequirementInfo={} %GIDa_178eee66_d6c3_4911_8a9b_fff821777d46  mask(SetNTC){}
      mask help: SetNTC library block
  BasAssiPahFwlFlt : simulink/Sources/Enumerated Constant  RequirementInfo={} %GIDa_acac850b_2127_4f9e_8633_f23729900187  OutDataTypeStr=Enum: NtcNr1  Value=NtcNr1.NTCNR_0X0D3  SampleTime=inf
  BaseAssistFwlReached : Subsystem  RequirementInfo={} %GIDa_6c312aa7_5aa7_43a9_8850_2eb3014894e2  mask(SetNTC){}
      mask help: SetNTC library block
  Constant1 : Constant  RequirementInfo={} %GIDa_39480dc0_09d1_43c3_833e_34f36c223161  Value=0  OutDataTypeStr=uint8
  Constant6 : Constant  RequirementInfo={} %GIDa_115e743d_71d8_4e1a_9d44_628f83cdb5d1  Value=0  OutDataTypeStr=uint8
  Constant8 : Constant  RequirementInfo={} %GIDa_8d0f4c58_4637_4c33_aff5_a7c1397682de  Value=0  OutDataTypeStr=uint8
  CopyRight2 : Subsystem  Description=|  mask(Copyright Information){none=on}
      | Copyright info block.                                               
      |                                                                     
      | Place copyright information at the top of every subsystem in design.
      mask prompts: none "No parameters"
      mask help: Place copyright information at the top of every subsystem in design.
      mask Display:
      | NxtrConf = 'Nexteer Confidential';
      | 
      | sys = bdroot; %handle for the current model ("system")
      | first = get_param(sys,'Created');
      | first = first(end-3:end);  %year is last four digits
      | 
      | last = get_param(sys,'LastModifiedDate');
      | if isempty(last)
      |     last = datestr(now,'yyyy');
      | else
      |     last = last(end-3:end);
      | end
      | 
      | if strcmp(first,last)
      |     fprintf('%s -- Copyright %s Nexteer',NxtrConf,first)
      | else
      |     fprintf('%s -- %s%s- %s Nexteer',NxtrConf,char(169),first,last)
      | end
  Enumerated Constant1 : simulink/Sources/Enumerated Constant  RequirementInfo={} %GIDa_7dd1537e_4f7d_4058_ab7f_7a927ea087ae  OutDataTypeStr=Enum: NtcSts1  Value=NtcSts1.NTCSTS_PASSD  SampleTime=inf
  Enumerated Constant4 : simulink/Sources/Enumerated Constant  RequirementInfo={} %GIDa_fd14c1c3_79c3_413d_be3c_1933ad90baa7  OutDataTypeStr=Enum: NtcSts1  Value=NtcSts1.NTCSTS_PASSD  SampleTime=inf
  Enumerated Constant5 : simulink/Sources/Enumerated Constant  RequirementInfo={} %GIDa_cfcbc4d2_3d6d_4cd1_96ef_00b438be0997  OutDataTypeStr=Enum: NtcSts1  Value=NtcSts1.NTCSTS_PASSD  SampleTime=inf
  FwlActvLpFilInit : Fil/FilLpInit  Ic=0  Ts=ARCHGLBPRM_2MILLISEC_SEC_F32  Freq=AssiPahFwlFwlActvLpFilFrq  StVar=FwlActvLpFilStVari
  Ground : Ground
  Ground1 : Ground
  Ground2 : Ground
  HiFrqAssiFwlReached : Subsystem  RequirementInfo={} %GIDa_a4d42b87_492f_4c2f_ad1c_3796a4d25afd  mask(SetNTC){}
      mask help: SetNTC library block
  HiFrqAssiPahFwlFlt : simulink/Sources/Enumerated Constant  RequirementInfo={} %GIDa_18e475c1_c348_49ea_9744_f9192fbc55d0  OutDataTypeStr=Enum: NtcNr1  Value=NtcNr1.NTCNR_0X0D2  SampleTime=inf
  HiFrqFilinit : Fil/FilLpInit  Ic=0  Ts=ARCHGLBPRM_2MILLISEC_SEC_F32  Freq=AssiPahFwlCmdSplitLpFilFrq  StVar=HiFrqCmdLpFilStVari
  LowrBndFilinit : Fil/FilLpInit  Ic=0  Ts=ARCHGLBPRM_2MILLISEC_SEC_F32  Freq=AssiPahFwlCmdSplitLpFilFrq  StVar=LowrLimLpFilStVari
  UpprBndFilinit : Fil/FilLpInit  Ic=0  Ts=ARCHGLBPRM_2MILLISEC_SEC_F32  Freq=AssiPahFwlCmdSplitLpFilFrq  StVar=UpprLimLpFilStVari
  wires:
  AssiFwlFlt/1 -> AssiFwlFltMode/1(NtcNr)
  Enumerated Constant4/1 -> AssiFwlFltMode/3(NtcSts)
  Ground/1 -> AssiFwlFltMode/4(DebStep)
  Constant1/1 -> AssiFwlFltMode/2(NtcStInfo)
  HiFrqAssiPahFwlFlt/1 -> HiFrqAssiFwlReached/1(NtcNr)
  Constant6/1 -> HiFrqAssiFwlReached/2(NtcStInfo)
  Enumerated Constant1/1 -> HiFrqAssiFwlReached/3(NtcSts)
  Ground1/1 -> HiFrqAssiFwlReached/4(DebStep)
  BasAssiPahFwlFlt/1 -> BaseAssistFwlReached/1(NtcNr)
  Constant8/1 -> BaseAssistFwlReached/2(NtcStInfo)
  Enumerated Constant5/1 -> BaseAssistFwlReached/3(NtcSts)
  Ground2/1 -> BaseAssistFwlReached/4(DebStep)

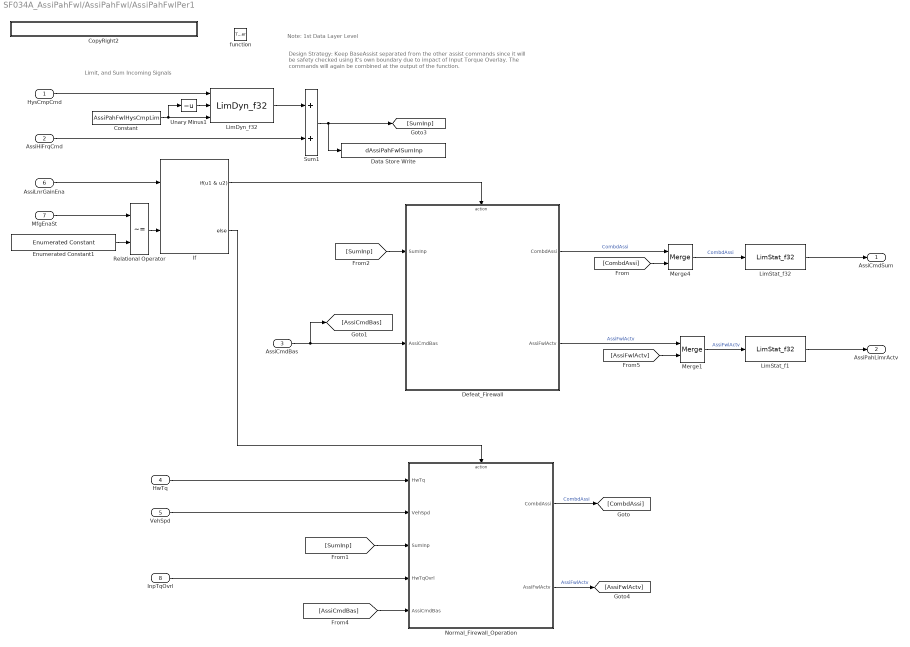
== system SF034A_AssiPahFwl/AssiPahFwl/AssiPahFwlPer1 ==
  note: Design Strategy:  Keep BaseAssist separated from the other assist commands since
      | it will be safety checked using it's own boundary due to impact of Input Torque Overlay.
      | The commands will again be combined at the output of the function.
  note: Limit, and Sum Incoming Signals
  note: Note: 1st Data Layer Level
  HysCmpCmd : Inport
  AssiHiFrqCmd : Inport  Port=2
  AssiCmdBas : Inport  Port=3
  HwTq : Inport  Port=4
  VehSpd : Inport  Port=5
  AssiLnrGainEna : Inport  Port=6
  MfgEnaSt : Inport  Port=7
  InpTqOvrl : Inport  Port=8
  function : TriggerPort  TriggerType=function-call
  Constant : Constant  RequirementInfo={} %GIDa_7d354adc_4d6b_482b_8452_7bb208e12ebc  Value=AssiPahFwlHysCmpLim
  CopyRight2 : Subsystem  Description=|  mask(Copyright Information){none=on}
      | Copyright info block.                                               
      |                                                                     
      | Place copyright information at the top of every subsystem in design.
      mask prompts: none "No parameters"
      mask help: Place copyright information at the top of every subsystem in design.
      mask Display:
      | NxtrConf = 'Nexteer Confidential';
      | 
      | sys = bdroot; %handle for the current model ("system")
      | first = get_param(sys,'Created');
      | first = first(end-3:end);  %year is last four digits
      | 
      | last = get_param(sys,'LastModifiedDate');
      | if isempty(last)
      |     last = datestr(now,'yyyy');
      | else
      |     last = last(end-3:end);
      | end
      | 
      | if strcmp(first,last)
      |     fprintf('%s -- Copyright %s Nexteer',NxtrConf,first)
      | else
      |     fprintf('%s -- %s%s- %s Nexteer',NxtrConf,char(169),first,last)
      | end
  Data Store Write : DataStoreWrite  DataStoreName=dAssiPahFwlSumInp
  Defeat_Firewall : Subsystem  TreatAsAtomicUnit=on
  Enumerated Constant1 : simulink/Sources/Enumerated Constant  RequirementInfo={} %GIDa_1b992b17_2365_4259_9dd8_ede73e4bb2d4  OutDataTypeStr=Enum: MfgEnaSt1  Value=MfgEnaSt1.MFGENAST_PRDNMOD  SampleTime=inf
  If : If  NumInputs=2  IfExpression=u1 & u2
  LimDyn_f32 : NxtrLim/LimDyn_f32
  LimStat_f1 : NxtrLim/LimStat_f32  LoLim=ASSIPAHLIMRACTVLOLIM_ULS_F32  HiLim=ASSIPAHLIMRACTVHILIM_ULS_F32
      settings: AttributesFormatString=|
      | Low Limit: %<LoLim>
      | High Limit:%<HiLim>
  LimStat_f32 : NxtrLim/LimStat_f32  LoLim=SYSGLBPRM_MOTTQCMDLOLIM_MOTNWTMTR_F32  HiLim=SYSGLBPRM_MOTTQCMDHILIM_MOTNWTMTR_F32
      settings: AttributesFormatString=|
      | Low Limit: %<LoLim>
      | High Limit:%<HiLim>
  Merge1 : Merge
  Merge4 : Merge
  Normal_Firewall_Operation : Subsystem  TreatAsAtomicUnit=on
  Relational Operator : RelationalOperator  Operator=~=  OutDataTypeStr=boolean
  Sum1 : Sum  SaturateOnIntegerOverflow=on  InputSameDT=on  OutDataTypeStr=Inherit: Same as first input
  Unary Minus1 : UnaryMinus
  AssiCmdSum : Outport
  AssiPahLimrActv : Outport  Port=2
  wires:
  HysCmpCmd/1 -> LimDyn_f32/1
  Merge1/1 -> LimStat_f1/1  "AssiFwlActv"
  VehSpd/1 -> Normal_Firewall_Operation/2(VehSpd)
  HwTq/1 -> Normal_Firewall_Operation/1(HwTq)
  Sum1/1 -> [SumInp], Data Store Write/1
  AssiLnrGainEna/1 -> If/1
  Defeat_Firewall/1(CombdAssi) -> Merge4/1  "CombdAssi"
  [SumInp] -> Normal_Firewall_Operation/3(SumInp)
  If/2 -> Normal_Firewall_Operation/Action
  Merge4/1 -> LimStat_f32/1  "CombdAssi"
  Defeat_Firewall/2(AssiFwlActv) -> Merge1/1  "AssiFwlActv"
  Normal_Firewall_Operation/2(AssiFwlActv) -> [AssiFwlActv]  "AssiFwlActv"
  Normal_Firewall_Operation/1(CombdAssi) -> [CombdAssi]  "CombdAssi"
  If/1 -> Defeat_Firewall/Action
  InpTqOvrl/1 -> Normal_Firewall_Operation/4(HwTqOvrl)
  AssiCmdBas/1 -> Defeat_Firewall/2(AssiCmdBas), [AssiCmdBas]
  [AssiCmdBas] -> Normal_Firewall_Operation/5(AssiCmdBas)
  LimDyn_f32/1 -> Sum1/1
  Constant/1 -> Unary Minus1/1, LimDyn_f32/3
  Unary Minus1/1 -> LimDyn_f32/2
  AssiHiFrqCmd/1 -> Sum1/2
  LimStat_f32/1 -> AssiCmdSum/1
  LimStat_f1/1 -> AssiPahLimrActv/1
  [CombdAssi] -> Merge4/2
  [AssiFwlActv] -> Merge1/2
  [SumInp] -> Defeat_Firewall/1(SumInp)
  Enumerated Constant1/1 -> Relational Operator/2
  Relational Operator/1 -> If/2
  MfgEnaSt/1 -> Relational Operator/1

== system SF034A_AssiPahFwl/AssiPahFwl/CopyRight2 ==

== system SF034A_AssiPahFwl/Init Call Simulation/CopyRight2 ==

== system SF034A_AssiPahFwl/AssiPahFwl/AssiPahFwlInit1/AssiFwlFltMode ==
  NtcNr : Inport
  NtcStInfo : Inport  Port=2
  NtcSts : Inport  Port=3
  DebStep : Inport  Port=4
  SetNtcSts : Subsystem  RequirementInfo={} %GIDa_110ade24_31e1_4802_ac8f_b2c4321f1444  TreatAsAtomicUnit=on
      settings: RTWSystemCode=Inline
  wires:
  NtcStInfo/1 -> SetNtcSts/2(NtcStInfo)
  DebStep/1 -> SetNtcSts/4(DebStep)
  NtcSts/1 -> SetNtcSts/3(NtcSts)
  NtcNr/1 -> SetNtcSts/1(NtcNr)  "NtcNr"

== system SF034A_AssiPahFwl/AssiPahFwl/AssiPahFwlInit1/BaseAssistFwlReached ==
  NtcNr : Inport
  NtcStInfo : Inport  Port=2
  NtcSts : Inport  Port=3
  DebStep : Inport  Port=4
  SetNtcSts : Subsystem  RequirementInfo={} %GIDa_77627834_42c7_48e3_8712_da98c3a0b740  TreatAsAtomicUnit=on
      settings: RTWSystemCode=Inline
  wires:
  NtcStInfo/1 -> SetNtcSts/2(NtcStInfo)
  DebStep/1 -> SetNtcSts/4(DebStep)
  NtcSts/1 -> SetNtcSts/3(NtcSts)
  NtcNr/1 -> SetNtcSts/1(NtcNr)  "NtcNr"

== system SF034A_AssiPahFwl/AssiPahFwl/AssiPahFwlInit1/CopyRight2 ==

== system SF034A_AssiPahFwl/AssiPahFwl/AssiPahFwlInit1/HiFrqAssiFwlReached ==
  NtcNr : Inport
  NtcStInfo : Inport  Port=2
  NtcSts : Inport  Port=3
  DebStep : Inport  Port=4
  SetNtcSts : Subsystem  RequirementInfo={} %GIDa_4eea81e2_7d1b_49d7_b5b8_cf0a80e6e5bc  TreatAsAtomicUnit=on
      settings: RTWSystemCode=Inline
  wires:
  NtcNr/1 -> SetNtcSts/1(NtcNr)  "NtcNr"
  NtcSts/1 -> SetNtcSts/3(NtcSts)
  DebStep/1 -> SetNtcSts/4(DebStep)
  NtcStInfo/1 -> SetNtcSts/2(NtcStInfo)

== system SF034A_AssiPahFwl/AssiPahFwl/AssiPahFwlPer1/CopyRight2 ==

== system SF034A_AssiPahFwl/AssiPahFwl/AssiPahFwlPer1/Defeat_Firewall ==
  SumInp : Inport
  AssiCmdBas : Inport  Port=2
  Action Port : ActionPort  ActionType=then
  Constant7 : Constant  Value=0  OutDataTypeStr=single
      settings: AttributesFormatString=%<OutDataTypeStr>
  CopyRight2 : Subsystem  Description=|  mask(Copyright Information){none=on}
      | Copyright info block.                                               
      |                                                                     
      | Place copyright information at the top of every subsystem in design.
      mask prompts: none "No parameters"
      mask help: Place copyright information at the top of every subsystem in design.
      mask Display:
      | NxtrConf = 'Nexteer Confidential';
      | 
      | sys = bdroot; %handle for the current model ("system")
      | first = get_param(sys,'Created');
      | first = first(end-3:end);  %year is last four digits
      | 
      | last = get_param(sys,'LastModifiedDate');
      | if isempty(last)
      |     last = datestr(now,'yyyy');
      | else
      |     last = last(end-3:end);
      | end
      | 
      | if strcmp(first,last)
      |     fprintf('%s -- Copyright %s Nexteer',NxtrConf,first)
      | else
      |     fprintf('%s -- %s%s- %s Nexteer',NxtrConf,char(169),first,last)
      | end
  Sum2 : Sum  SaturateOnIntegerOverflow=on  InputSameDT=on  OutDataTypeStr=Inherit: Same as first input
  CombdAssi : Outport
  AssiFwlActv : Outport  Port=2
  wires:
  Constant7/1 -> AssiFwlActv/1
  SumInp/1 -> Sum2/1
  AssiCmdBas/1 -> Sum2/2
  Sum2/1 -> CombdAssi/1

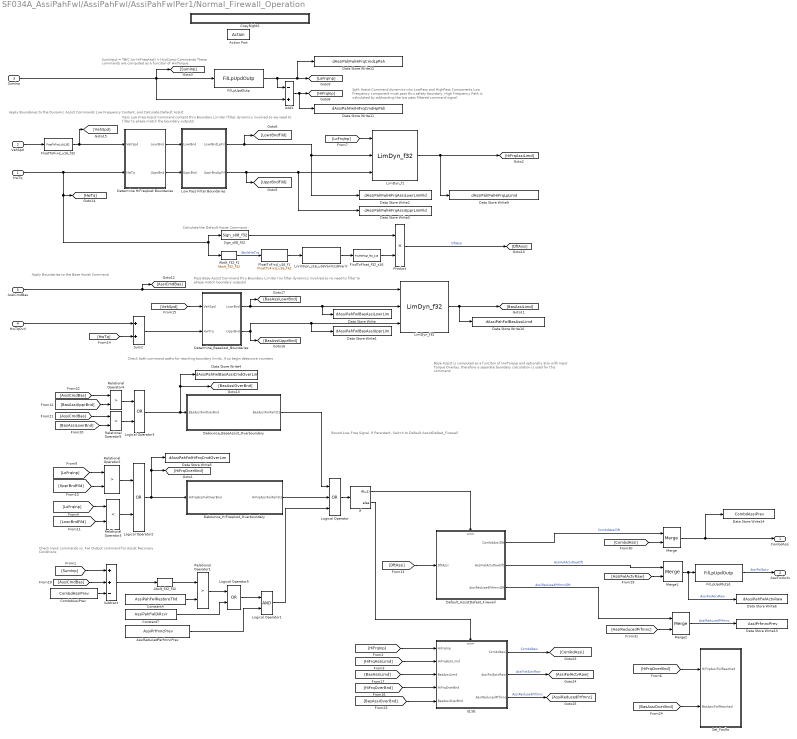
== system SF034A_AssiPahFwl/AssiPahFwl/AssiPahFwlPer1/Normal_Firewall_Operation ==
  note: Apply Boundaries to the Base Assist Command
  note: Bound Low-Freq Signal. If Persistent, Switch to Default AssistDefeat_Firewall
  note: Check both command paths for reaching boundary limits, if so begin debounce counters
  note: Split Assist Command dynamics into LowPass and HighPass Components
      | Low Frequency component must pass thru safety boundary.  High Frequency
      | Path is calculated by subtracting the low pass filtered command signal.
  note: Pass Base Assist Command thru Boundary Limiter (no filter dynamics involved so no need to filter to phase match boundary outputs)
  note: Pass Low Freq Assist Command content thru Boundary Limiter (filter dynamics involved so we need to filter to phase match the boundary outputs)
  note: SumInput = TBIC (or HiFreqAsst) + HysComp Commands
      | These commands are computed as a funciton of HwTorque
  note: Base Assist is computed as a funciton of HwTorque and optionally also
      | with Input Torque Overlay, therefore a separate boundary calculation is
      | used for this command.
  note: Apply Boundaries to the Dynamic Assist Commands Low Frequency Content, and Calculate Default Assist
  note: Calculate the Default Assist Command
  note: Check Input commands vs. Fwl Output command for
      | Assist Recovery Conditions
  HwTq : Inport
  VehSpd : Inport  Port=2
  SumInp : Inport  Port=3
  HwTqOvrl : Inport  Port=4
  AssiCmdBas : Inport  Port=5
  Action Port : ActionPort  ActionType=else
  Abslt_f32_f1 : NxtrAbslt/Abslt_f32_f32  SFunctionSpec=single y1 = Abslt_f32_f32(single u1)
      settings: AttributesFormatString=%<Name>
  Abslt_f32_f32 : NxtrAbslt/Abslt_f32_f32  SFunctionSpec=single y1 = Abslt_f32_f32(single u1)
      settings: AttributesFormatString=%<Name>
  Add1 : Sum  Inputs=-+
  AssiReducedPerfmncPrev : DataStoreRead  DataStoreName=AssiPrfmncPrev
  CombdAssiPrev : DataStoreRead  DataStoreName=CombdAssiPrev
  Constant4 : Constant  Value=AssiPahFwlRestoreThd
  Constant7 : Constant  Value=AssiPahFwlDiRcvr  OutDataTypeStr=boolean
  CopyRight2 : Subsystem  Description=|  mask(Copyright Information){none=on}
      | Copyright info block.                                               
      |                                                                     
      | Place copyright information at the top of every subsystem in design.
      mask prompts: none "No parameters"
      mask help: Place copyright information at the top of every subsystem in design.
      mask Display:
      | NxtrConf = 'Nexteer Confidential';
      | 
      | sys = bdroot; %handle for the current model ("system")
      | first = get_param(sys,'Created');
      | first = first(end-3:end);  %year is last four digits
      | 
      | last = get_param(sys,'LastModifiedDate');
      | if isempty(last)
      |     last = datestr(now,'yyyy');
      | else
      |     last = last(end-3:end);
      | end
      | 
      | if strcmp(first,last)
      |     fprintf('%s -- Copyright %s Nexteer',NxtrConf,first)
      | else
      |     fprintf('%s -- %s%s- %s Nexteer',NxtrConf,char(169),first,last)
      | end
  Data Store Write : DataStoreWrite  DataStoreName=dAssiPahFwlBasAssiLowrLim
  Data Store Write1 : DataStoreWrite  DataStoreName=dAssiPahFwlBasAssiUpprLim
  Data Store Write10 : DataStoreWrite  DataStoreName=dAssiPahFwlBasAssiLimd
  Data Store Write11 : DataStoreWrite  DataStoreName=dAssiPahFwlHiFrqCmdHpPah
  Data Store Write12 : DataStoreWrite  DataStoreName=dAssiPahFwlHiFrqCmdLpPah
  Data Store Write13 : DataStoreWrite  DataStoreName=AssiPrfmncPrev
  Data Store Write14 : DataStoreWrite  DataStoreName=CombdAssiPrev
  Data Store Write2 : DataStoreWrite  DataStoreName=dAssiPahFwlHiFrqAssiLowrLimFild
  Data Store Write3 : DataStoreWrite  DataStoreName=dAssiPahFwlHiFrqAssiUpprLimFild
  Data Store Write4 : DataStoreWrite  DataStoreName=dAssiPahFwlBasAssiCmdOverLim
  Data Store Write5 : DataStoreWrite  DataStoreName=dAssiPahFwlHiFrqCmdOverLim
  Data Store Write6 : DataStoreWrite  DataStoreName=dAssiPahFwlActvRaw
  Data Store Write9 : DataStoreWrite  DataStoreName=dAssiPahFwlHiFrqLpLimd
  Debounce_BaseAssist_Overboundary : Subsystem
  Debounce_HiFreqAsst_Overboundary : Subsystem
  Default_AssistDefeat_Firewall : Subsystem  TreatAsAtomicUnit=on
  Determine HiFreqAsst Boundaries : Subsystem
  Determine_BaseAsst_Boundaries : Subsystem
  ELSE : Subsystem  TreatAsAtomicUnit=on
  FilLpUpdOutp : Fil/FilLpUpdOutp  StVar=HiFrqCmdLpFilStVari
      settings: AttributesFormatString=StVar: %<StVar>
  FilLpUpdOutp1 : Fil/FilLpUpdOutp  StVar=FwlActvLpFilStVari
      settings: AttributesFormatString=StVar: %<StVar>
  FixdToFloat_f32_s16 : FixdToFloat/FixdToFloat_f32_s16  Param1=11
  FloatToFixd_u16_f1 : FloatToFixd/FloatToFixd_u16_f32  Param1=8
  FloatToFixd_u16_f32 : FloatToFixd/FloatToFixd_u16_f32  Param1=7
  If : If  IfExpression=u1
  LimDyn_f1 : NxtrLim/LimDyn_f32
  LimDyn_f32 : NxtrLim/LimDyn_f32
  LnrIntrpn_s16_u16VariXs16VariY : LnrIntrpn/LnrIntrpn_s16_u16VariXs16VariY  XTbl=AssiPahFwlDftAssiX  YTbl=AssiPahFwlDftAssiY
      settings: AttributesFormatString=Lnr ( u16VariX , s16VariY )
  Logical Operator : Logic  Operator=OR  Inputs=3  AllPortsSameDT=off  OutDataTypeStr=boolean
  Logical Operator1 : Logic  AllPortsSameDT=off  OutDataTypeStr=boolean
  Logical Operator2 : Logic  Operator=OR  AllPortsSameDT=off  OutDataTypeStr=boolean
  Logical Operator3 : Logic  Operator=OR  AllPortsSameDT=off  OutDataTypeStr=boolean
  Logical Operator5 : Logic  Operator=OR  AllPortsSameDT=off  OutDataTypeStr=boolean
  Low Pass Filter Boundaries : Subsystem
  Merge : Merge
  Merge1 : Merge
  Merge2 : Merge
  Product : Product  RndMeth=Zero
  Relational Operator1 : RelationalOperator  Operator=>  OutDataTypeStr=boolean
  Relational Operator2 : RelationalOperator  Operator=>  OutDataTypeStr=boolean
  Relational Operator3 : RelationalOperator  Operator=<  OutDataTypeStr=boolean
  Relational Operator4 : RelationalOperator  Operator=>  OutDataTypeStr=boolean
  Relational Operator5 : RelationalOperator  Operator=<  OutDataTypeStr=boolean
  Set_Faults : Subsystem
  Sign_s08_f32 : NxtrSign/Sign_s08_f32  SFunctionSpec=int8 y1 = Sign_s08_f32(single u1)
  Subtract : Sum  Inputs=++-
  Sum2 : Sum  SaturateOnIntegerOverflow=on  InputSameDT=on  OutDataTypeStr=Inherit: Same as first input
  CombdAssi : Outport
  AssiFwlActv : Outport  Port=2
  wires:
  FilLpUpdOutp1/1 -> AssiFwlActv/1  "AssiFwlActv"
  [LoFrqInp] -> LimDyn_f1/1
  Debounce_HiFreqAsst_Overboundary/1(HiFrqAssiFwlFailSts) -> Logical Operator/2
  Abslt_f32_f1/1 -> FloatToFixd_u16_f1/1  "AbsltHwTrq"
  LimDyn_f1/1 -> Data Store Write9/1, [HiFrqAssiLimd]
  Subtract/1 -> Abslt_f32_f32/1
  Abslt_f32_f32/1 -> Relational Operator1/1
  Constant4/1 -> Relational Operator1/2
  Logical Operator/1 -> If/1
  Logical Operator1/1 -> Logical Operator/3
  FixdToFloat_f32_s16/1 -> Product/2
  [LoFrqInp] -> Relational Operator2/1
  [LoFrqInp] -> Relational Operator3/1
  Relational Operator2/1 -> Logical Operator2/1
  Relational Operator3/1 -> Logical Operator2/2
  [UpprBndFild] -> Relational Operator2/2
  [LowrBndFild] -> Relational Operator3/2
  AssiReducedPerfmncPrev/1 -> Logical Operator1/2
  If/1 -> Default_AssistDefeat_Firewall/Action
  If/2 -> ELSE/Action
  Product/1 -> [DftAssi]  "DftAssi"
  [DftAssi] -> Default_AssistDefeat_Firewall/1(DftAssi)
  Merge1/1 -> Data Store Write6/1, FilLpUpdOutp1/1  "AssiFwlActvRaw"
  Merge2/1 -> Data Store Write13/1  "AssiReducedPrfmnc"
  SumInp/1 -> Add1/2, FilLpUpdOutp/1, [SumInp]
  [SumInp] -> Subtract/1
  Logical Operator2/1 -> Debounce_HiFreqAsst_Overboundary/1(HiFrqAssiFwlOverBnd), Data Store Write5/1, [HiFrqOverBnd]
  [HwTq] -> Sum2/2
  LimDyn_f32/1 -> Data Store Write10/1, [BasAssiLimd]
  Sum2/1 -> Determine_BaseAsst_Boundaries/2(HwTrq)
  HwTqOvrl/1 -> Sum2/1
  [VehSpd] -> Determine_BaseAsst_Boundaries/1(VehSpd)
  FilLpUpdOutp/1 -> Add1/1, [LoFrqInp], Data Store Write12/1
  AssiCmdBas/1 -> [AssiCmdBas], LimDyn_f32/1
  [AssiCmdBas] -> Subtract/2
  [AssiCmdBas] -> Relational Operator4/1
  [AssiCmdBas] -> Relational Operator5/1
  Relational Operator4/1 -> Logical Operator3/1
  Relational Operator5/1 -> Logical Operator3/2
  [BasAssiUpprBnd] -> Relational Operator4/2
  [BasAssiLowrBnd] -> Relational Operator5/2
  Logical Operator3/1 -> Debounce_BaseAssist_Overboundary/1(BasAssiFwlOverBnd), Data Store Write4/1, [BasAssiOverBnd]
  Determine_BaseAsst_Boundaries/1(LowrBnd) -> [BasAssiLowrBnd], Data Store Write/1, LimDyn_f32/2
  Determine_BaseAsst_Boundaries/2(UpprBnd) -> Data Store Write1/1, LimDyn_f32/3, [BasAssiUpprBnd]
  Sign_s08_f32/1 -> Product/1
  FloatToFixd_u16_f1/1 -> LnrIntrpn_s16_u16VariXs16VariY/1
  LnrIntrpn_s16_u16VariXs16VariY/1 -> FixdToFloat_f32_s16/1
  HwTq/1 -> [HwTq], Abslt_f32_f1/1, Sign_s08_f32/1, Determine HiFreqAsst Boundaries/2(HwTq)
  VehSpd/1 -> FloatToFixd_u16_f32/1
  [HiFrqOverBnd] -> Set_Faults/1(HiFrqAssiFwlReached)
  [BasAssiOverBnd] -> Set_Faults/2(BasAssiFwlReached)
  Add1/1 -> Data Store Write11/1, [HiFrqInp]
  Determine HiFreqAsst Boundaries/1(LowrBnd) -> Low Pass Filter Boundaries/1(LowrBnd)
  Determine HiFreqAsst Boundaries/2(UpprBnd) -> Low Pass Filter Boundaries/2(UpprBnd)
  Low Pass Filter Boundaries/1(LowrBndLpFil) -> Data Store Write2/1, LimDyn_f1/2, [LowrBndFild]
  Low Pass Filter Boundaries/2(UpprBndLpFil) -> Data Store Write3/1, LimDyn_f1/3, [UpprBndFild]
  Debounce_BaseAssist_Overboundary/1(BasAssiFwlFailSts) -> Logical Operator/1
  Logical Operator5/1 -> Logical Operator1/1
  Relational Operator1/1 -> Logical Operator5/1
  Constant7/1 -> Logical Operator5/2
  Default_AssistDefeat_Firewall/1(CombdAssiDft) -> Merge/1  "CombdAssiDft"
  Default_AssistDefeat_Firewall/2(AssiFwlActvRawDft) -> Merge1/1  "AssiFwlActvRawDft"
  Default_AssistDefeat_Firewall/3(AssiReducedPrfmncDft) -> Merge2/1  "AssiReducedPrfmncDft"
  ELSE/2(AssiFwlActvRaw) -> [AssiFwlActvRaw]  "AssiFwlActvRaw"
  ELSE/1(CombdAssi) -> [CombdAssi]  "CombdAssi"
  [CombdAssi] -> Merge/2
  ELSE/3(AssiReducedPrfmnc) -> [AssiReducedPrfmnc]  "AssiReducedPrfmnc"
  [AssiReducedPrfmnc] -> Merge2/2
  [AssiFwlActvRaw] -> Merge1/2
  Merge/1 -> CombdAssi/1, Data Store Write14/1
  CombdAssiPrev/1 -> Subtract/3
  [HiFrqAssiLimd] -> ELSE/2(HiFrqAssiLimd)
  [HiFrqInp] -> ELSE/1(HiFrqInp)
  [BasAssiLimd] -> ELSE/3(BasAssiLimd)
  [BasAssiOverBnd] -> ELSE/5(BasAssiOverBnd)
  [HiFrqOverBnd] -> ELSE/4(HiFrqOverBnd)
  FloatToFixd_u16_f32/1 -> [VehSpd], Determine HiFreqAsst Boundaries/1(VehSpd)

== system SF034A_AssiPahFwl/AssiPahFwl/AssiPahFwlInit1/AssiFwlFltMode/SetNtcSts ==
  note: Note:
      |
      | - "ISO Fault Debounce Design" Simulink block intent to use here for Simulation purpose only. Do not Code this block
  NtcNr : Inport
  NtcStInfo : Inport  Port=2
  NtcSts : Inport  Port=3
  DebStep : Inport  Port=4
  CopyRight2 : Subsystem  Description=|  mask(Copyright Information){none=on}
      | Copyright info block.                                               
      |                                                                     
      | Place copyright information at the top of every subsystem in design.
      mask prompts: none "No parameters"
      mask help: Place copyright information at the top of every subsystem in design.
      mask Display:
      | NxtrConf = 'Nexteer Confidential';
      | 
      | sys = bdroot; %handle for the current model ("system")
      | first = get_param(sys,'Created');
      | if(isempty(first))
      |     first = datestr(now,'yyyy');
      | else
      |     first = first(end-3:end);  %year is last four digits
      | end
      | 
      | last = get_param(sys,'LastModifiedDate');
      | if isempty(last)
      |     last = datestr(now,'yyyy');
      | else
      |     last = last(end-3:end);
      | end
      | 
      | if strcmp(first,last)
      |     fprintf('%s -- Copyright %s Nexteer',NxtrConf,first)
      | else
      |     fprintf('%s -- %s%s- %s Nexteer',NxtrConf,char(169),first,last)
      | end
  Data Store Write : DataStoreWrite  DataStoreName=Ntc0x0C9Qlfr
  Data Type Conversion : DataTypeConversion  OutDataTypeStr=Enum: SigQlfr1
  Ground : Ground
  ISO Fault Debounce Design : Stateflow chart  TreatAsAtomicUnit=on
      settings: AttributesFormatString=|
      | Simulation Purpose Only.
      | Do Not Code this block
      | Diagnostic Manager Owns this requirement
  Terminator : Terminator
  Terminator1 : Terminator
  wires:
  Ground/1 -> ISO Fault Debounce Design/3(SvcClr)
  ISO Fault Debounce Design/1(Qualifier) -> Data Type Conversion/1
  DebStep/1 -> ISO Fault Debounce Design/2(DebStep)
  NtcNr/1 -> Terminator/1
  NtcStInfo/1 -> Terminator1/1
  NtcSts/1 -> ISO Fault Debounce Design/1(NtcSts)
  Data Type Conversion/1 -> Data Store Write/1

== system SF034A_AssiPahFwl/AssiPahFwl/AssiPahFwlInit1/BaseAssistFwlReached/SetNtcSts ==
  note: Note:
      |
      | - "ISO Fault Debounce Design" Simulink block intent to use here for Simulation purpose only. Do not Code this block
  NtcNr : Inport
  NtcStInfo : Inport  Port=2
  NtcSts : Inport  Port=3
  DebStep : Inport  Port=4
  CopyRight2 : Subsystem  Description=|  mask(Copyright Information){none=on}
      | Copyright info block.                                               
      |                                                                     
      | Place copyright information at the top of every subsystem in design.
      mask prompts: none "No parameters"
      mask help: Place copyright information at the top of every subsystem in design.
      mask Display:
      | NxtrConf = 'Nexteer Confidential';
      | 
      | sys = bdroot; %handle for the current model ("system")
      | first = get_param(sys,'Created');
      | if(isempty(first))
      |     first = datestr(now,'yyyy');
      | else
      |     first = first(end-3:end);  %year is last four digits
      | end
      | 
      | last = get_param(sys,'LastModifiedDate');
      | if isempty(last)
      |     last = datestr(now,'yyyy');
      | else
      |     last = last(end-3:end);
      | end
      | 
      | if strcmp(first,last)
      |     fprintf('%s -- Copyright %s Nexteer',NxtrConf,first)
      | else
      |     fprintf('%s -- %s%s- %s Nexteer',NxtrConf,char(169),first,last)
      | end
  Data Store Write : DataStoreWrite  DataStoreName=Ntc0x0D3Qlfr
  Data Type Conversion : DataTypeConversion  OutDataTypeStr=Enum: SigQlfr1
  Ground : Ground
  ISO Fault Debounce Design : Stateflow chart  TreatAsAtomicUnit=on
      settings: AttributesFormatString=|
      | Simulation Purpose Only.
      | Do Not Code this block
      | Diagnostic Manager Owns this requirement
  Terminator : Terminator
  Terminator1 : Terminator
  wires:
  Ground/1 -> ISO Fault Debounce Design/3(SvcClr)
  ISO Fault Debounce Design/1(Qualifier) -> Data Type Conversion/1
  DebStep/1 -> ISO Fault Debounce Design/2(DebStep)
  NtcNr/1 -> Terminator/1
  NtcStInfo/1 -> Terminator1/1
  NtcSts/1 -> ISO Fault Debounce Design/1(NtcSts)
  Data Type Conversion/1 -> Data Store Write/1

== system SF034A_AssiPahFwl/AssiPahFwl/AssiPahFwlInit1/HiFrqAssiFwlReached/SetNtcSts ==
  note: Note:
      |
      | - "ISO Fault Debounce Design" Simulink block intent to use here for Simulation purpose only. Do not Code this block
  NtcNr : Inport
  NtcStInfo : Inport  Port=2
  NtcSts : Inport  Port=3
  DebStep : Inport  Port=4
  CopyRight2 : Subsystem  Description=|  mask(Copyright Information){none=on}
      | Copyright info block.                                               
      |                                                                     
      | Place copyright information at the top of every subsystem in design.
      mask prompts: none "No parameters"
      mask help: Place copyright information at the top of every subsystem in design.
      mask Display:
      | NxtrConf = 'Nexteer Confidential';
      | 
      | sys = bdroot; %handle for the current model ("system")
      | first = get_param(sys,'Created');
      | if(isempty(first))
      |     first = datestr(now,'yyyy');
      | else
      |     first = first(end-3:end);  %year is last four digits
      | end
      | 
      | last = get_param(sys,'LastModifiedDate');
      | if isempty(last)
      |     last = datestr(now,'yyyy');
      | else
      |     last = last(end-3:end);
      | end
      | 
      | if strcmp(first,last)
      |     fprintf('%s -- Copyright %s Nexteer',NxtrConf,first)
      | else
      |     fprintf('%s -- %s%s- %s Nexteer',NxtrConf,char(169),first,last)
      | end
  Data Store Write : DataStoreWrite  DataStoreName=Ntc0x0D2Qlfr
  Data Type Conversion : DataTypeConversion  OutDataTypeStr=Enum: SigQlfr1
  Ground : Ground
  ISO Fault Debounce Design : Stateflow chart  TreatAsAtomicUnit=on
      settings: AttributesFormatString=|
      | Simulation Purpose Only.
      | Do Not Code this block
      | Diagnostic Manager Owns this requirement
  Terminator : Terminator
  Terminator1 : Terminator
  wires:
  Data Type Conversion/1 -> Data Store Write/1
  NtcSts/1 -> ISO Fault Debounce Design/1(NtcSts)
  NtcStInfo/1 -> Terminator1/1
  NtcNr/1 -> Terminator/1
  DebStep/1 -> ISO Fault Debounce Design/2(DebStep)
  ISO Fault Debounce Design/1(Qualifier) -> Data Type Conversion/1
  Ground/1 -> ISO Fault Debounce Design/3(SvcClr)

== system SF034A_AssiPahFwl/AssiPahFwl/AssiPahFwlPer1/Defeat_Firewall/CopyRight2 ==

== system SF034A_AssiPahFwl/AssiPahFwl/AssiPahFwlPer1/Normal_Firewall_Operation/CopyRight2 ==
